simulink model "menabtrigsubsys"  (Simulink 8.0)
settings: Solver=FixedStepDiscrete  StartTime=0.0  StopTime=10.0  FixedStep=1  RelTol=1e-3
settings Model: Creator=mtocci  LastModifiedBy=mtocci
settings DataIOCC: LimitDataPoints=off  SaveFormat=StructureWithTime  SignalLoggingSaveFormat=ModelDataLogs
settings OptimizationCC: InlineParams=on
settings DebuggingCC: FcnCallInpInsideContextMsg=Use local settings  StrictBusMsg=ErrorOnBusTreatedAsVector
settings GRTTargetCC: CombineOutputUpdateFcns=off

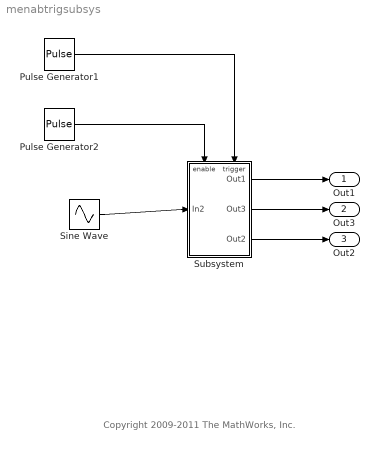
== system menabtrigsubsys ==
  note: Copyright 2009-2011 The MathWorks, Inc.
  Pulse Generator1 : DiscretePulseGenerator  Amplitude=[1 1 2 2]
  Pulse Generator2 : DiscretePulseGenerator  Amplitude=int8([2 2 1 1])  Period=3  PhaseDelay=1
  Sine Wave : Sin  SineType=Sample based  Samples=5  SampleTime=1
  Subsystem : Subsystem
  Out1 : Outport  InitialOutput=0
  Out3 : Outport  Port=2  InitialOutput=0
  Out2 : Outport  Port=3  InitialOutput=0
  wires:
  Subsystem/1(Out1) -> Out1/1
  Subsystem/2(Out3) -> Out3/1
  Sine Wave/1 -> Subsystem/1(In2)
  Pulse Generator2/1 -> Subsystem/Enable
  Subsystem/3(Out2) -> Out2/1
  Pulse Generator1/1 -> Subsystem/Trigger

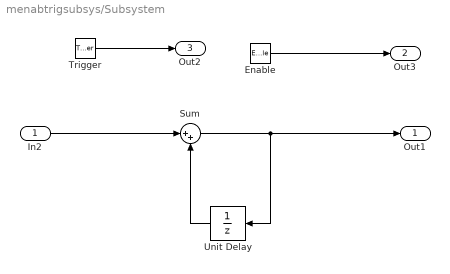
== system menabtrigsubsys/Subsystem ==
  In2 : Inport
  Enable : EnablePort  ShowOutputPort=on
  Trigger : TriggerPort  ShowOutputPort=on
  Sum : Sum  Inputs=|++
  Unit Delay : UnitDelay  SampleTime=-1
  Out1 : Outport  InitialOutput=0
  Out3 : Outport  Port=2  InitialOutput=0
  Out2 : Outport  Port=3  InitialOutput=0
  wires:
  In2/1 -> Sum/1
  Sum/1 -> Out1/1, Unit Delay/1
  Unit Delay/1 -> Sum/2
  Enable/1 -> Out3/1
  Trigger/1 -> Out2/1
